simulink model "dodavanje_estimatora_2012"  (R2016a)
settings: Solver=ode45  StartTime=0.0  StopTime=20000.0  RelTol=1e-12  AbsTol=1e-9
undefined symbols (not defined in the file): Al, Bl, Cl, d1, d2, d3, h0, h10, h20, h30, hmax, K, kd, L, Ld, q0, r, s, sout, Ts
settings Model: Creator=Vukan  LastModifiedBy=Moon Raven
settings DataIOCC: SaveFormat=StructureWithTime
settings OptimizationCC: LifeSpan=10
settings DebuggingCC: FcnCallInpInsideContextMsg=EnableAllAsWarning  SFUnexpectedBacktrackingDiag=error  SFNoUnconditionalDefaultTransitionDiag=error
settings HardwareCC: ProdWordSize=32  ProdHWDeviceType=Specified
settings GRTTargetCC: TargetLangStandard=C99 (ISO)  GeneratePreprocessorConditionals=Use local settings
settings ConfigComp: CovMetricSettings=dwe  CovHtmlReporting=off  CovSaveCumulativeToWorkspaceVar=off  CovSaveSingleToWorkspaceVar=off  CovExternalEMLEnable=on

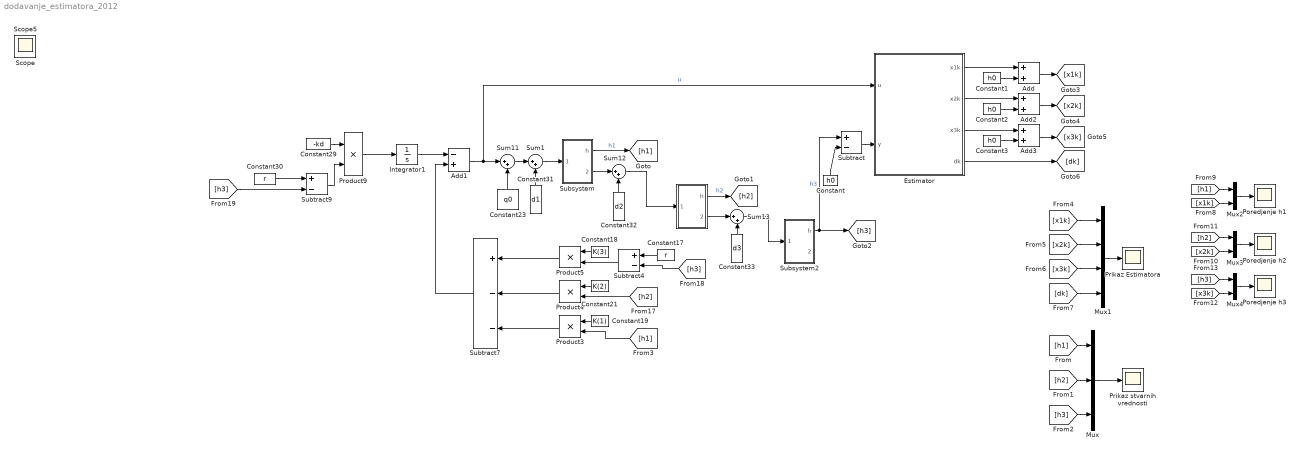
== system dodavanje_estimatora_2012 ==
  " " : Subsystem
  Add : Sum
  Add1 : Sum  Inputs=-+
  Add2 : Sum
  Add3 : Sum
  Constant{,1..3} (4 alike) : Constant  Value=h0
  Constant17 : Constant  Value=r
  Constant18 : Constant  Value=K(3)
  Constant19 : Constant  Value=K(1)
  Constant21 : Constant  Value=K(2)
  Constant23 : Constant  Value=q0
  Constant29 : Constant  Value=-kd
  Constant30 : Constant  Value=r
  Constant31 : Constant  Value=d1
  Constant32 : Constant  Value=d2
  Constant33 : Constant  Value=d3
  Estimator : MATLAB Function  TreatAsAtomicUnit=on
  Integrator1 : Integrator
  Mux : Mux  Inputs=3
  Mux1 : Mux
  Mux2 : Mux  Inputs=2
  Mux3 : Mux  Inputs=2
  Mux4 : Mux  Inputs=2
  Poredjenje h1 : Scope
  Poredjenje h2 : Scope
  Poredjenje h3 : Scope
  Prikaz Estimatora : Scope
  Prikaz stvarnih vrednosti : Scope
  Product{3..5,9} (4 alike) : Product
  Subsystem : Subsystem
  Subsystem2 : Subsystem
  Subtract : Sum  Inputs=+-
  Subtract4 : Sum  Inputs=+-
  Subtract7 : Sum  Inputs=+--
  Subtract9 : Sum  Inputs=+-
  Sum{1,11..13} (4 alike) : Sum  Inputs=|++
  Scope : Scope
  Scope5 : Scope
  wires:
  Subsystem/1(h) -> [h1]  "h1"
  " "/1(h) -> [h2]  "h2"
  Subsystem2/1(h) -> Subtract/1, [h3]  "h3"
  Mux/1 -> Prikaz stvarnih vrednosti/1
  [h1] -> Mux/1
  [h2] -> Mux/2
  [h3] -> Mux/3
  Constant19/1 -> Product3/1
  Constant21/1 -> Product4/1
  Constant18/1 -> Product5/1
  Product3/1 -> Subtract7/3
  Product4/1 -> Subtract7/2
  Product5/1 -> Subtract7/1
  Constant23/1 -> Sum11/2
  Add1/1 -> Estimator/1(u), Sum11/1  "u"
  Constant29/1 -> Product9/1
  Subtract9/1 -> Product9/2
  Constant30/1 -> Subtract9/1
  [h3] -> Subtract9/2
  Product9/1 -> Integrator1/1
  Integrator1/1 -> Add1/1
  Sum1/1 -> Subsystem/1(qin)
  Constant31/1 -> Sum1/2
  Sum11/1 -> Sum1/1
  Constant32/1 -> Sum12/2
  Sum12/1 -> " "/1(qin)
  Subsystem/2(qout) -> Sum12/1
  " "/2(qout) -> Sum13/1
  Sum13/1 -> Subsystem2/1(qin)
  Constant33/1 -> Sum13/2
  [h2] -> Product4/2
  [h1] -> Product3/2
  Subtract4/1 -> Product5/2
  [h3] -> Subtract4/2
  Constant17/1 -> Subtract4/1
  Subtract7/1 -> Add1/2
  Estimator/4(dk) -> [dk]
  [x1k] -> Mux1/1
  [x2k] -> Mux1/2
  [x3k] -> Mux1/3
  [dk] -> Mux1/4
  Mux1/1 -> Prikaz Estimatora/1
  Subtract/1 -> Estimator/2(y)
  Constant/1 -> Subtract/2
  Add/1 -> [x1k]
  Estimator/1(x1k) -> Add/1
  Add2/1 -> [x2k]
  Add3/1 -> [x3k]
  Estimator/2(x2k) -> Add2/1
  Estimator/3(x3k) -> Add3/1
  Constant1/1 -> Add/2
  Constant2/1 -> Add2/2
  Constant3/1 -> Add3/2
  Mux2/1 -> Poredjenje h1/1
  Mux3/1 -> Poredjenje h2/1
  Mux4/1 -> Poredjenje h3/1
  [x1k] -> Mux2/2
  [h1] -> Mux2/1
  [h2] -> Mux3/1
  [x2k] -> Mux3/2
  [h3] -> Mux4/1
  [x3k] -> Mux4/2

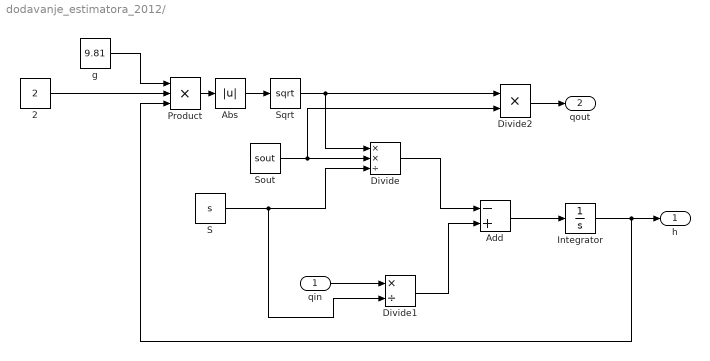
== system dodavanje_estimatora_2012/  ==
  qin : Inport
  2 : Constant  Value=2
  Abs : Abs
  Add : Sum  Inputs=-+
  Divide : Product  Inputs=**/
  Divide1 : Product  Inputs=*/
  Divide2 : Product  Inputs=**
  Integrator : Integrator  InitialCondition=h20  LimitOutput=on  UpperSaturationLimit=hmax  LowerSaturationLimit=0
  Product : Product  Inputs=3
  "S " : Constant  Value=s
  Sout : Constant  Value=sout
  Sqrt : Sqrt  SaturateOnIntegerOverflow=on
  g : Constant  Value=9.81
  h : Outport
  qout : Outport  Port=2
  wires:
  Divide2/1 -> qout/1
  Integrator/1 -> Product/3, h/1
  Abs/1 -> Sqrt/1
  Product/1 -> Abs/1
  2/1 -> Product/2
  Sqrt/1 -> Divide/1, Divide2/1
  Divide1/1 -> Add/2
  g/1 -> Product/1
  Add/1 -> Integrator/1
  qin/1 -> Divide1/1
  Divide/1 -> Add/1
  "S "/1 -> Divide/3, Divide1/2
  Sout/1 -> Divide/2, Divide2/2

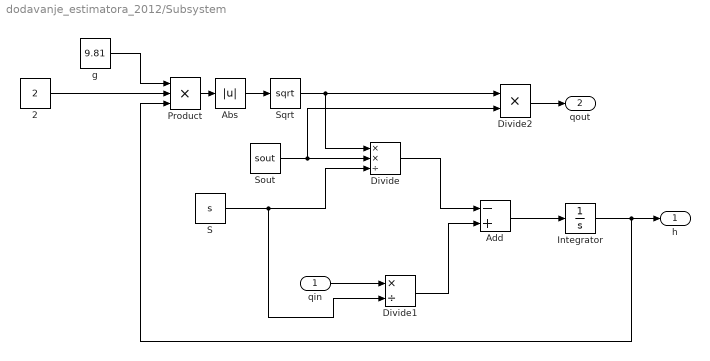
== system dodavanje_estimatora_2012/Subsystem ==
  qin : Inport
  2 : Constant  Value=2
  Abs : Abs
  Add : Sum  Inputs=-+
  Divide : Product  Inputs=**/
  Divide1 : Product  Inputs=*/
  Divide2 : Product  Inputs=**
  Integrator : Integrator  InitialCondition=h10  LimitOutput=on  UpperSaturationLimit=hmax  LowerSaturationLimit=0
  Product : Product  Inputs=3
  "S " : Constant  Value=s
  Sout : Constant  Value=sout
  Sqrt : Sqrt  SaturateOnIntegerOverflow=on
  g : Constant  Value=9.81
  h : Outport
  qout : Outport  Port=2
  wires:
  Sout/1 -> Divide2/2, Divide/2
  "S "/1 -> Divide1/2, Divide/3
  Divide/1 -> Add/1
  qin/1 -> Divide1/1
  Add/1 -> Integrator/1
  g/1 -> Product/1
  Divide1/1 -> Add/2
  Sqrt/1 -> Divide2/1, Divide/1
  2/1 -> Product/2
  Product/1 -> Abs/1
  Abs/1 -> Sqrt/1
  Integrator/1 -> h/1, Product/3
  Divide2/1 -> qout/1

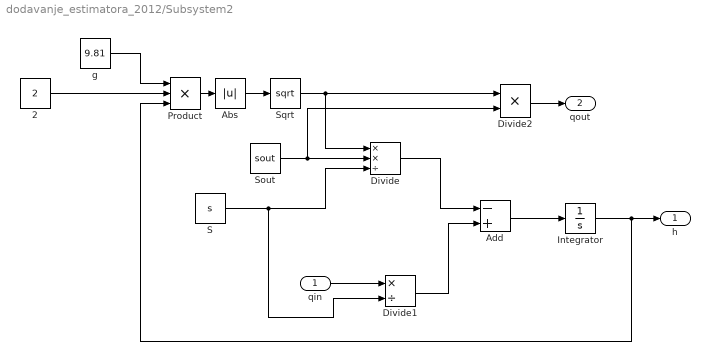
== system dodavanje_estimatora_2012/Subsystem2 ==
  qin : Inport
  2 : Constant  Value=2
  Abs : Abs
  Add : Sum  Inputs=-+
  Divide : Product  Inputs=**/
  Divide1 : Product  Inputs=*/
  Divide2 : Product  Inputs=**
  Integrator : Integrator  InitialCondition=h30  LimitOutput=on  UpperSaturationLimit=hmax  LowerSaturationLimit=0
  Product : Product  Inputs=3
  "S " : Constant  Value=s
  Sout : Constant  Value=sout
  Sqrt : Sqrt  SaturateOnIntegerOverflow=on
  g : Constant  Value=9.81
  h : Outport
  qout : Outport  Port=2
  wires:
  Sout/1 -> Divide2/2, Divide/2
  "S "/1 -> Divide1/2, Divide/3
  Divide/1 -> Add/1
  qin/1 -> Divide1/1
  Add/1 -> Integrator/1
  g/1 -> Product/1
  Divide1/1 -> Add/2
  Sqrt/1 -> Divide2/1, Divide/1
  2/1 -> Product/2
  Product/1 -> Abs/1
  Abs/1 -> Sqrt/1
  Integrator/1 -> h/1, Product/3
  Divide2/1 -> qout/1

== matlab function dodavanje_estimatora_2012/Estimator ==
  settings: updateMethod=DISCRETE  sampleTime=Ts
  data: u input; x1k output; y input; x2k output; x3k output; dk output; Al parameter; Bl parameter; Ts parameter; L parameter; Ld parameter; Cl parameter
function [x1k,x2k,x3k,dk] = estimator(u, y, Al, Bl, Ts, L, Ld, Cl)

persistent xk;
if isempty(xk)
    xk = [0 0 0]';
end
persistent dkk;
if isempty(dkk)
    dkk = 0;
end


dkk_new = dkk + Ts*Ld*(y - Cl*xk);
xk_new = xk + Ts*(Al*xk + Bl*dkk + Bl*u + L*(y-Cl*xk));

dkk = dkk_new;
xk = xk_new;

x1k = xk(1);
x2k = xk(2);
x3k = xk(3);
dk = dkk;
